simulink model "ex4"  (R2015a)
settings: Solver=ode45  StartTime=0.0  StopTime=10.0  RelTol=1e-3
undefined symbols (not defined in the file): g, l
libraries: simulink x1
settings Model: Creator=fschalle  LastModifiedBy=fschalle

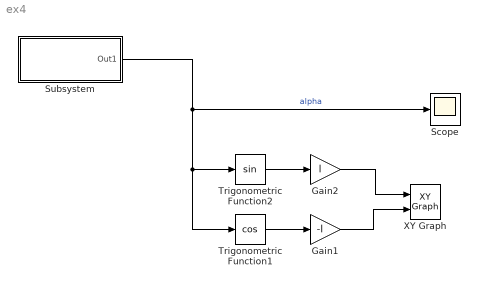
== system ex4 ==
  Gain1 : Gain  Gain=-l
  Gain2 : Gain  Gain=l
  Scope : Scope
  Subsystem : Subsystem
  Trigonometric Function1 : Trigonometry  Operator=cos
  Trigonometric Function2 : Trigonometry
  XY Graph : simulink/Sinks/XY Graph  xmin=-5  xmax=5  ymin=-5  ymax=5  st=-1
  wires:
  Trigonometric Function1/1 -> Gain1/1
  Trigonometric Function2/1 -> Gain2/1
  Gain1/1 -> XY Graph/2
  Gain2/1 -> XY Graph/1
  Subsystem/1(Out1) -> Trigonometric Function1/1, Trigonometric Function2/1, Scope/1  "alpha"

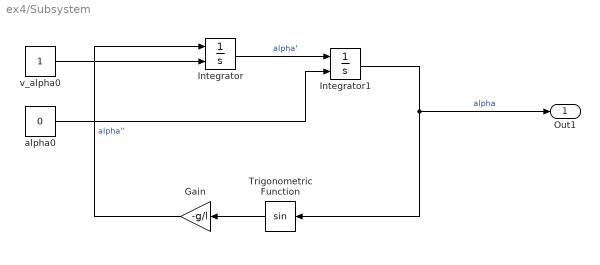
== system ex4/Subsystem ==
  Gain : Gain  Gain=-g/l
  Integrator : Integrator  InitialConditionSource=external
  Integrator1 : Integrator  InitialConditionSource=external
  Trigonometric Function : Trigonometry
  "alpha0 " : Constant  Value=0
  "v_alpha0 " : Constant
  Out1 : Outport
  wires:
  Integrator/1 -> Integrator1/1  "alpha'"
  "v_alpha0 "/1 -> Integrator/2
  Trigonometric Function/1 -> Gain/1
  Gain/1 -> Integrator/1  "alpha''"
  "alpha0 "/1 -> Integrator1/2
  Integrator1/1 -> Trigonometric Function/1, Out1/1  "alpha"
